simulink model "HEVPlant_Ptbs_V1b_18a"  (R2018b)
settings: configuration reference "Config_Plant" (kept outside this file)
PreLoadFcn:
  | HEVPlant_Ptbs_V1_BusInfo
undefined symbols (not defined in the file or in its folder): b_axle, b_driveshaft, DiffRatio, EngDriveRatio, k_axle, k_driveshaft, MotGbRatio, RWheel
libraries: autolibshared x4, autolibsharedcoupling x2, autolibshareddiff x1, simulink x1, autolibdatasheetbattery x1
(part 1 of 3)
settings Model: DataDictionary=HEVPlant_Ptbs_V1.sldd  OrderedModelArguments=off  Creator=IAEC Nishito  LastModifiedBy=E00026

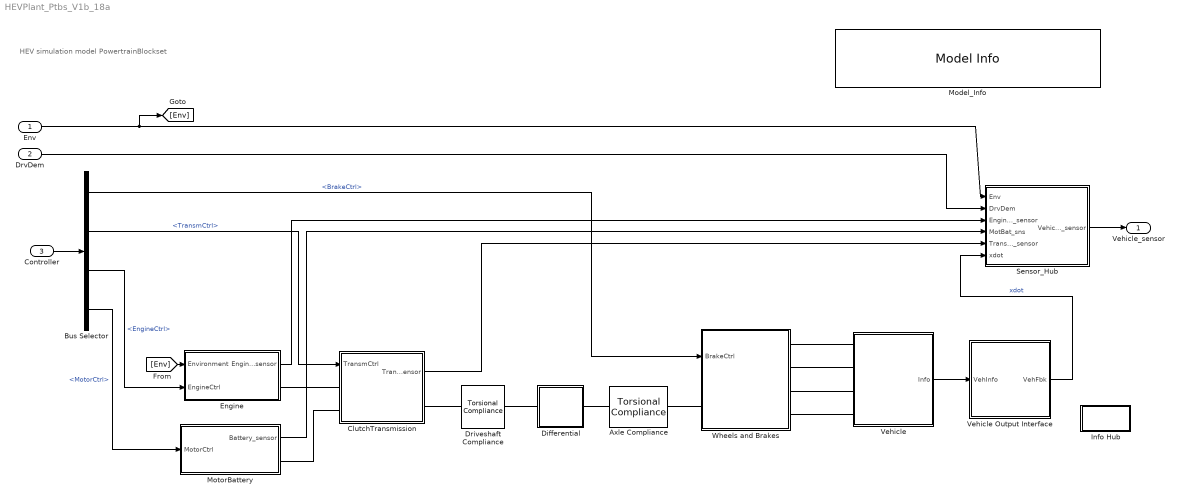
== system HEVPlant_Ptbs_V1b_18a ==
  note: HEV simulation model
      | PowertrainBlockset
  Env : Inport  OutDataTypeStr=Bus: Environment_Bus
  DrvDem : Inport  Port=2  OutDataTypeStr=Bus: Driver_demand_Bus
  Controller : Inport  Port=3  OutDataTypeStr=Bus: Ctrl_intg_Bus
      settings: AttributesFormatString=%<OutDataTypeStr>
  Axle Compliance : autolibsharedcoupling/Torsional Compliance  port_config=Two-way connection  k=k_axle  b=b_axle  theta_o=0  domega_o=0  omega_c=wc_shaft  blkID=0  aMode=1
      settings: SourceProductName=Powertrain Blockset  SourceProductBaseCode=PW
  Bus Selector : BusSelector  OutputSignals=BrakeCtrl,TransmCtrl,EngineCtrl,MotorCtrl
  ClutchTransmission : Subsystem
  Differential : Subsystem
  Driveshaft Compliance : autolibsharedcoupling/Torsional Compliance  port_config=Two-way connection  k=k_driveshaft  b=b_driveshaft  theta_o=0  domega_o=0  omega_c=wc_shaft  blkID=0  aMode=1
      settings: SourceProductName=Powertrain Blockset  SourceProductBaseCode=PW
  Engine : Subsystem
  Info Hub : Subsystem
  Model_Info : simulink/Model-Wide Utilities/Model Info  Frame=on  DisplayStringWithTags=|  HorizontalTextAlignment=Left  LeftAlignmentValue=0.02
      | Version  %<ModelVersion>
      | LastModifided by %<LastModifiedBy>  Date %<LastModificationDate>
      | Description  %<Description>
  MotorBattery : Subsystem
  Sensor_Hub : Subsystem
  Vehicle : Subsystem
  Vehicle Output Interface : Subsystem
  Wheels and Brakes : Subsystem
  Vehicle_sensor : Outport  OutDataTypeStr=Bus: Vehicle_sensor_Bus  VectorParamsAs1DForOutWhenUnconnected=off
      settings: AttributesFormatString=%<OutDataTypeStr>
  wires:
  Controller/1 -> Bus Selector/1
  Env/1 -> [Env], Sensor_Hub/1(Env)
  DrvDem/1 -> Sensor_Hub/2(DrvDem)
  Bus Selector/1 -> Wheels and Brakes/1(BrakeCtrl)  "<BrakeCtrl>"
  Vehicle/1(Info) -> Vehicle Output Interface/1(VehInfo)
  Bus Selector/4 -> MotorBattery/1(MotorCtrl)  "<MotorCtrl>"
  Bus Selector/2 -> ClutchTransmission/1(TransmCtrl)  "<TransmCtrl>"
  Bus Selector/3 -> Engine/2(EngineCtrl)  "<EngineCtrl>"
  Vehicle Output Interface/1(VehFbk) -> Sensor_Hub/6(xdot)  "xdot"
  MotorBattery/1(Battery_sensor) -> Sensor_Hub/4(MotBat_sns)
  Sensor_Hub/1(Vehicle_sensor) -> Vehicle_sensor/1
  ClutchTransmission/1(Transm_sensor) -> Sensor_Hub/5(Transm_sensor)
  Engine/1(Engine_sensor) -> Sensor_Hub/3(Engine_sensor)
  [Env] -> Engine/1(Environment)
  connections:
  Wheels and Brakes/RConn2 -- Vehicle/LConn2
  Vehicle/LConn1 -- Wheels and Brakes/RConn1
  Wheels and Brakes/RConn4 -- Vehicle/LConn4
  Wheels and Brakes/RConn3 -- Vehicle/LConn3
  Axle Compliance/RConn1 -- Wheels and Brakes/LConn1
  Axle Compliance/LConn1 -- Differential/RConn1
  Driveshaft Compliance/RConn1 -- Differential/LConn1
  Driveshaft Compliance/LConn1 -- ClutchTransmission/RConn1
  Engine/RConn1 -- ClutchTransmission/LConn1
  MotorBattery/RConn1 -- ClutchTransmission/LConn2

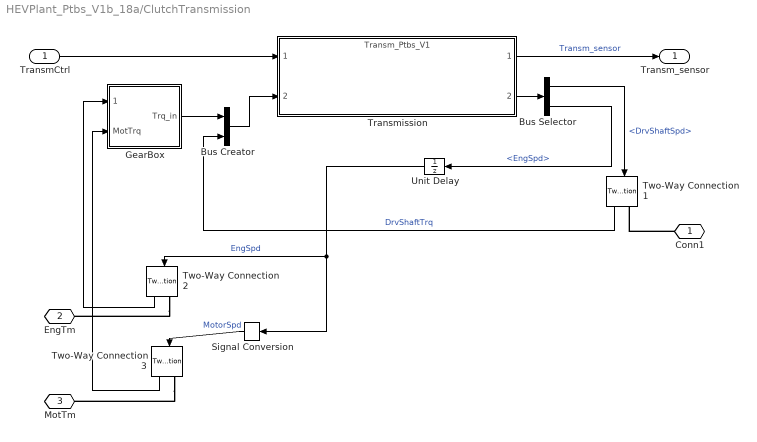
== system HEVPlant_Ptbs_V1b_18a/ClutchTransmission ==
  TransmCtrl : Inport
  Bus Creator : BusCreator  Inputs=2
  Bus Selector : BusSelector  OutputSignals=DrvShaftSpd,EngSpd
  GearBox : Subsystem
  Signal Conversion : SignalConversion  OverrideOpt=off
  Transmission : ModelReference  ModelNameDialog=Transm_Ptbs_V1.slx  SimulationMode=Normal  ModelReferenceVersion=1.52
  Two-Way Connection1 : TwoWayConnection
  Two-Way Connection2 : TwoWayConnection
  Two-Way Connection3 : TwoWayConnection
  Unit Delay : UnitDelay  SampleTime=-1  HasFrameUpgradeWarning=on
  Conn1 : PMIOPort  Side=Right
  EngTm : PMIOPort  Port=2  Side=Left
  MotTm : PMIOPort  Port=3  Side=Left
  Transm_sensor : Outport  VectorParamsAs1DForOutWhenUnconnected=off
  wires:
  Two-Way Connection3/1 -> GearBox/2(MotTrq)
  Two-Way Connection2/1 -> GearBox/1(EngineTrq)
  Signal Conversion/1 -> Two-Way Connection3/1  "MotorSpd"
  TransmCtrl/1 -> Transmission/1
  GearBox/1(Trq_in) -> Bus Creator/1
  Two-Way Connection1/1 -> Bus Creator/2  "DrvShaftTrq"
  Transmission/1 -> Transm_sensor/1  "Transm_sensor"
  Transmission/2 -> Bus Selector/1
  Bus Selector/1 -> Two-Way Connection1/1  "<DrvShaftSpd>"
  Bus Selector/2 -> Unit Delay/1  "<EngSpd>"
  Bus Creator/1 -> Transmission/2
  Unit Delay/1 -> Two-Way Connection2/1, Signal Conversion/1  "EngSpd"
  connections:
  Conn1/RConn1 -- Two-Way Connection1/RConn1
  Two-Way Connection2/RConn1 -- EngTm/RConn1
  Two-Way Connection3/RConn1 -- MotTm/RConn1

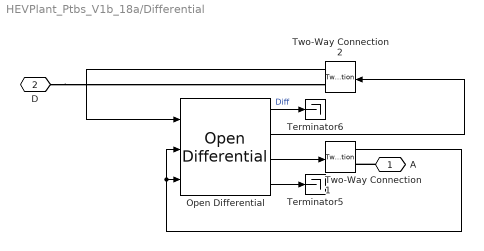
== system HEVPlant_Ptbs_V1b_18a/Differential ==
  Open Differential : autolibshareddiff/Open Differential  shaftSwitchMask=To the left of center-line  Ndiff=DiffRatio  Jd=.025  bd=1e-3  Jw1=.01  bw1=1e-3  Jw2=.01  bw2=1e-3  omegaw1o=0  omegaw2o=0  maxAbsSpd=5e3  aMode=1
      settings: SourceProductName=Powertrain Blockset  SourceProductBaseCode=PW
  Terminator5 : Terminator
  Terminator6 : Terminator
  Two-Way Connection1 : TwoWayConnection
  Two-Way Connection2 : TwoWayConnection
  A : PMIOPort  Side=Right
  D : PMIOPort  Port=2  Side=Left
  wires:
  Open Differential/3 -> Two-Way Connection1/1
  Open Differential/4 -> Terminator5/1
  Open Differential/1 -> Terminator6/1  "Diff"
  Open Differential/2 -> Two-Way Connection2/1
  Two-Way Connection1/1 -> Open Differential/2, Open Differential/3
  Two-Way Connection2/1 -> Open Differential/1
  connections:
  A/RConn1 -- Two-Way Connection1/RConn1
  D/RConn1 -- Two-Way Connection2/RConn1

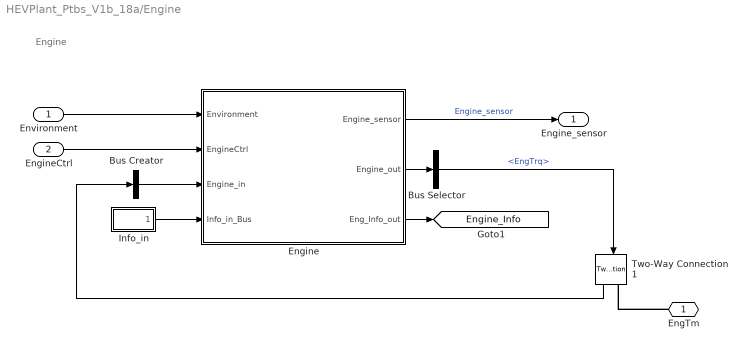
== system HEVPlant_Ptbs_V1b_18a/Engine ==
  note: Engine
  Environment : Inport
  EngineCtrl : Inport  Port=2
  Bus Creator : BusCreator  Inputs=1
  Bus Selector : BusSelector  OutputSignals=EngTrq
  Engine : Subsystem  Variant=on
  Info_in : Subsystem
  Two-Way Connection1 : TwoWayConnection
  EngTm : PMIOPort  Side=Right
  Engine_sensor : Outport  VectorParamsAs1DForOutWhenUnconnected=off
  tag scope: Engine_Info=global
  wires:
  Two-Way Connection1/1 -> Bus Creator/1
  Bus Selector/1 -> Two-Way Connection1/1  "<EngTrq>"
  Environment/1 -> Engine/1("Environment ")
  EngineCtrl/1 -> Engine/2(EngineCtrl)
  Bus Creator/1 -> Engine/3("Engine_in ")
  Info_in/1(Info_in) -> Engine/4("Info_in_Bus ")
  Engine/1(" Engine_sensor") -> Engine_sensor/1  "Engine_sensor"
  Engine/2(" Engine_out") -> Bus Selector/1
  Engine/3(" Eng_Info_out") -> [Engine_Info]
  connections:
  EngTm/RConn1 -- Two-Way Connection1/RConn1

== system HEVPlant_Ptbs_V1b_18a/Info Hub ==
  Terminator1 : Terminator
  wires:
  [Engine_Info] -> Terminator1/1

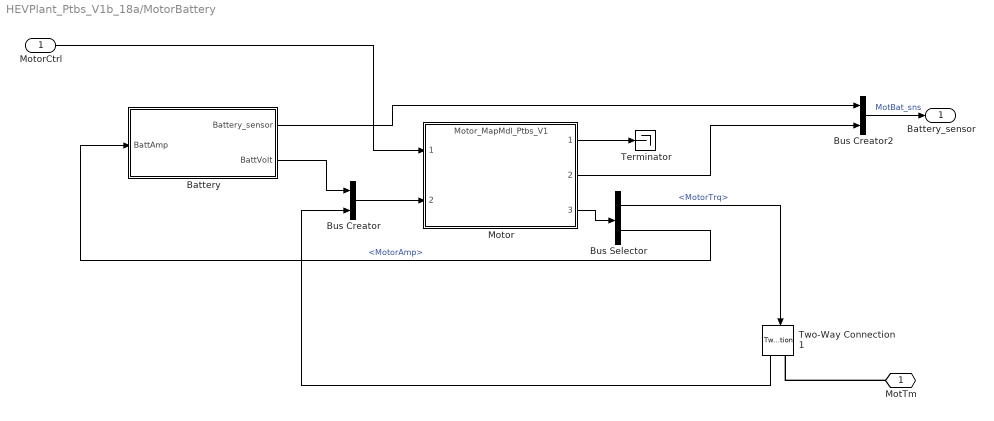
== system HEVPlant_Ptbs_V1b_18a/MotorBattery ==
  MotorCtrl : Inport
  Battery : Subsystem  TreatAsAtomicUnit=on
  Bus Creator : BusCreator  Inputs=2
  Bus Creator2 : BusCreator  Inputs=2
  Bus Selector : BusSelector  OutputSignals=MotorTrq,MotorAmp
  Motor : ModelReference  ModelNameDialog=Motor_MapMdl_Ptbs_V1  SimulationMode=Normal  ModelReferenceVersion=1.1343
  Terminator : Terminator
  Two-Way Connection1 : TwoWayConnection
  MotTm : PMIOPort  Side=Right
  Battery_sensor : Outport  VectorParamsAs1DForOutWhenUnconnected=off
  wires:
  Bus Creator2/1 -> Battery_sensor/1  "MotBat_sns"
  MotorCtrl/1 -> Motor/1
  Two-Way Connection1/1 -> Bus Creator/2
  Motor/2 -> Bus Creator2/2
  Battery/1(Battery_sensor) -> Bus Creator2/1
  Battery/2(BattVolt) -> Bus Creator/1
  Motor/3 -> Bus Selector/1
  Bus Selector/1 -> Two-Way Connection1/1  "<MotorTrq>"
  Bus Selector/2 -> Battery/1(BattAmp)  "<MotorAmp>"
  Motor/1 -> Terminator/1
  Bus Creator/1 -> Motor/2
  connections:
  MotTm/RConn1 -- Two-Way Connection1/RConn1

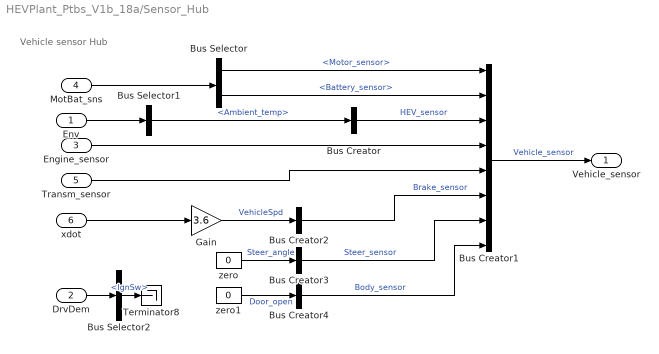
== system HEVPlant_Ptbs_V1b_18a/Sensor_Hub ==
  note: Vehicle sensor Hub
  Env : Inport
  DrvDem : Inport  Port=2
  Engine_sensor : Inport  Port=3
  MotBat_sns : Inport  Port=4
  Transm_sensor : Inport  Port=5
  xdot : Inport  Port=6
  Bus Creator : BusCreator  Inputs=1  OutDataTypeStr=Bus: HEV_sensor_Bus
      settings: AttributesFormatString=%<OutDataTypeStr>
  Bus Creator1 : BusCreator  Inputs=8  OutDataTypeStr=Bus:Vehicle_sensor_Bus
      settings: AttributesFormatString=%<OutDataTypeStr>
  Bus Creator2 : BusCreator  Inputs=1  OutDataTypeStr=Bus: Brake_sensor_Bus
      settings: AttributesFormatString=%<OutDataTypeStr>
  Bus Creator3 : BusCreator  Inputs=1  OutDataTypeStr=Bus: Steer_sensor_Bus
      settings: AttributesFormatString=%<OutDataTypeStr>
  Bus Creator4 : BusCreator  Inputs=1  OutDataTypeStr=Bus: Body_sensor_Bus
      settings: AttributesFormatString=%<OutDataTypeStr>
  Bus Selector : BusSelector  OutputSignals=Motor_sensor,Battery_sensor
  Bus Selector1 : BusSelector  OutputSignals=Ambient_temp
  Bus Selector2 : BusSelector  OutputSignals=IgnSw
  Gain : Gain  Gain=3.6
  Terminator8 : Terminator
  zero : Constant  Value=0
  zero1 : Constant  Value=0
  Vehicle_sensor : Outport  VectorParamsAs1DForOutWhenUnconnected=off
      settings: AttributesFormatString=%<OutDataTypeStr>
  wires:
  Bus Creator1/1 -> Vehicle_sensor/1  "Vehicle_sensor"
  Engine_sensor/1 -> Bus Creator1/4
  xdot/1 -> Gain/1
  MotBat_sns/1 -> Bus Selector/1
  Bus Selector/1 -> Bus Creator1/1  "<Motor_sensor>"
  Bus Selector/2 -> Bus Creator1/2  "<Battery_sensor>"
  Bus Creator/1 -> Bus Creator1/3  "HEV_sensor"
  Transm_sensor/1 -> Bus Creator1/5
  Gain/1 -> Bus Creator2/1  "VehicleSpd"
  Bus Creator2/1 -> Bus Creator1/6  "Brake_sensor"
  zero/1 -> Bus Creator3/1  "Steer_angle"
  zero1/1 -> Bus Creator4/1  "Door_open"
  Bus Creator3/1 -> Bus Creator1/7  "Steer_sensor"
  Bus Creator4/1 -> Bus Creator1/8  "Body_sensor"
  DrvDem/1 -> Bus Selector2/1
  Env/1 -> Bus Selector1/1
  Bus Selector1/1 -> Bus Creator/1  "<Ambient_temp>"
  Bus Selector2/1 -> Terminator8/1  "<IgnSw>"

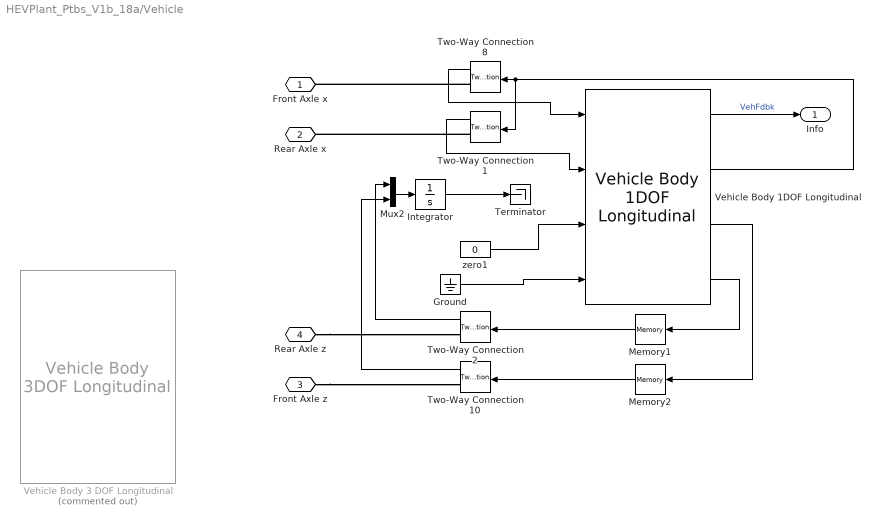
== system HEVPlant_Ptbs_V1b_18a/Vehicle ==
  Ground : Ground
  Integrator : Integrator
  Memory1 : Memory
  Memory2 : Memory
  Mux2 : Mux  Inputs=2
  Terminator : Terminator
  Two-Way Connection{1..2,8,10} (4 alike) : TwoWayConnection
  Vehicle Body 1DOF Longitudinal : autolibshared/Vehicle Body 1DOF Longitudinal  VariantControl=SL  aMode=1  NF=2  NR=2  m=1.723200000000000e+03  a=1.56  b=1.22  h=.5  Cd=.29  Af=2.27  x_o=0  xdot_o=0  Pabs=101325  T=273  g=9.81
      settings: SourceProductName=Powertrain Blockset  SourceProductBaseCode=PW
  Vehicle Body 3 DOF Longitudinal : autolibshared/Vehicle Body 3DOF Longitudinal  Commented=on  VariantControl=SL  groundType=Axle displacement, velocity  aMode=aMode  NF=2  NR=2  m=1.723200000000000e+03  a=1.56  b=1.22  h=.5  Cd=.29  Af=2.27  x_o=0  xdot_o=0  Cl=.1  z_o=-.35  zdot_o=0  Iyy=3000  Cpm=.1  theta_o=0  q_o=0  FskF=[-50, -1, 0, 2, 3, 52].*1.25e4  dzsF=[-5e-3, -1e-4, 0, .2, .2001, .2051]  FsbF=[-10000 -100 -10 0 10 100 10000]  dzdotsF=[-10 -1 -.1 0 .1 1 10]  FskR=[-50, -1, 0, 2, 3, 52].*7.5e3  dzsR=[-5e-3, -1e-4, 0, .2, .2001, .2051]  FsbR=[-10000 -100 -10 0 10 100 10000]  dzdotsR=[-10 -1 -.1 0 .1 1 10]  Pabs=101325  T=273  g=9.81  blkID=0
      settings: SourceProductName=Powertrain Blockset  SourceProductBaseCode=PW
  zero1 : Constant  Value=0
  Front Axle x : PMIOPort  Side=Left
  Rear Axle x : PMIOPort  Port=2  Side=Left
  Front Axle z : PMIOPort  Port=3  Side=Left
  Rear Axle z : PMIOPort  Port=4  Side=Left
  Info : Outport  VectorParamsAs1DForOutWhenUnconnected=off
  wires:
  Vehicle Body 1DOF Longitudinal/3 -> Memory2/1
  Two-Way Connection8/1 -> Vehicle Body 1DOF Longitudinal/1
  Vehicle Body 1DOF Longitudinal/1 -> Info/1  "VehFdbk"
  Ground/1 -> Vehicle Body 1DOF Longitudinal/4
  Two-Way Connection1/1 -> Vehicle Body 1DOF Longitudinal/2
  Vehicle Body 1DOF Longitudinal/4 -> Memory1/1
  Two-Way Connection2/1 -> Mux2/1
  Two-Way Connection10/1 -> Mux2/2
  Mux2/1 -> Integrator/1
  Integrator/1 -> Terminator/1
  zero1/1 -> Vehicle Body 1DOF Longitudinal/3
  Vehicle Body 1DOF Longitudinal/2 -> Two-Way Connection1/1, Two-Way Connection8/1
  Memory1/1 -> Two-Way Connection2/1
  Memory2/1 -> Two-Way Connection10/1
  connections:
  Two-Way Connection8/RConn1 -- Front Axle x/RConn1
  Front Axle z/RConn1 -- Two-Way Connection10/RConn1
  Two-Way Connection1/RConn1 -- Rear Axle x/RConn1
  Rear Axle z/RConn1 -- Two-Way Connection2/RConn1

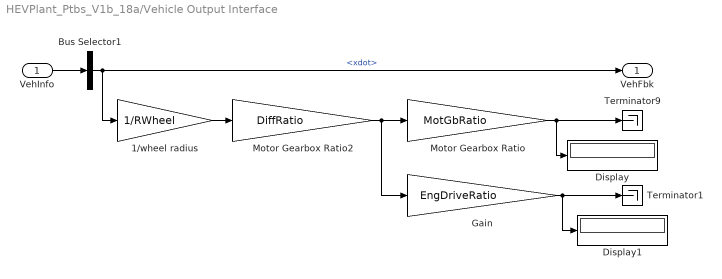
== system HEVPlant_Ptbs_V1b_18a/Vehicle Output Interface ==
  VehInfo : Inport
  1/wheel radius : Gain  Gain=1/RWheel
  Bus Selector1 : BusSelector  OutputSignals=BdyFrm.Cg.Vel.xdot
  Display : Display
  Display1 : Display
  Gain : Gain  Gain=EngDriveRatio
  Motor Gearbox Ratio : Gain  Gain=MotGbRatio
  Motor Gearbox Ratio2 : Gain  Gain=DiffRatio
  Terminator1 : Terminator
  Terminator9 : Terminator
  VehFbk : Outport  VectorParamsAs1DForOutWhenUnconnected=off
  wires:
  Bus Selector1/1 -> VehFbk/1, 1/wheel radius/1  "<xdot>"
  Gain/1 -> Display1/1, Terminator1/1
  Motor Gearbox Ratio/1 -> Display/1, Terminator9/1
  VehInfo/1 -> Bus Selector1/1
  Motor Gearbox Ratio2/1 -> Gain/1, Motor Gearbox Ratio/1
  1/wheel radius/1 -> Motor Gearbox Ratio2/1
